simulink model "Control_Test"  (R2020a)
settings: Solver=ode1  StartTime=0.0  StopTime=inf  FixedStep=0.001  RelTol=1e-3
InitFcn:
  | COM_config;
  | IO_config;
values from neighbouring files (symbols this model uses):
  AirDensity_kgpm3 = 1.225    [vehicle_controller.mat]
  BatteryCapacity_Wh = 83    [vehicle_controller.mat]
  BatteryInitialEnergy = 58.1    [vehicle_controller.mat]
  BatteryMaxVoltage_V = 96    [vehicle_controller.mat]
  BatteryVoltageCoefficient_x = [0 0.1 0.2 0.3 0.4 0.5 0.6 0.7 0.8 0.9 1]    [vehicle_controller.mat]
  BatteryVoltageCoefficient_y = [0.833333333333 0.85 0.866666666667 0.883333333333 0.9 0.916666666667 0.933333333333 0.95 0.966666666667 0.983333333333 1]    [vehicle_controller.mat]
  BodyInitialSpeed_mps = 0    [vehicle_controller.mat]
  BodyMass_kg = 900    [vehicle_controller.mat]
  CombustionEngineMaxTorque_Nm = 100    [vehicle_controller.mat]
  DragArea_m2 = 4.5    [vehicle_controller.mat]
  DragCoeficient_1 = 0.4    [vehicle_controller.mat]
  FrictionCoefficient_Nsprad = 0.01    [vehicle_controller.mat]
  GearboxRatio_0_1 = 3    [vehicle_controller.mat]
  Ke = 0.1178    [vehicle_controller.mat]
  Kt = 0.668    [vehicle_controller.mat]
  L = looptransfer.Lo    [H_infinity_control_design.m]    (also in LoopShaping.m = G*K; Vehicle_Car_Controller.m = P * C)
  R = 0.141176    [vehicle_controller.mat]
  WheelDiameter_m = 0.5    [vehicle_controller.mat]
undefined symbols (not defined in the file or in its folder): AI_01_range, AI_02_range, AI_03_range, AI_04_range, AI_05_range, AI_06_range, AO_01_max, AO_02_max, AO_03_max, AO_04_max, AO_05_max, AO_06_max, Battery_Voltage_Req, DI_01_mode, DI_01_pullUpDown, DI_02_mode, DI_02_pullUpDown, DI_03_mode, DI_03_pullUpDown, DI_04_mode, DI_04_pullUpDown, DI_05_mode, DI_05_pullUpDown, DI_06_mode, DI_06_pullUpDown, DI_vref_threshold, DO_01_mode, DO_01_outStage, DO_02_mode, DO_02_outStage, DO_03_mode, DO_03_outStage, DO_04_mode, DO_04_outStage, DO_05_mode, DO_05_outStage, DO_06_mode, DO_06_outStage, DO_vref_high, package_period, Serial_Port, Standard_Devices
libraries: simulink x8, sldrtlib x2, simulink_extras x1
(part 1 of 2)
settings Model: SimulationMode=external  Creator=matti  LastModifiedBy=matti
settings SolverCC: DecoupledContinuousIntegration=on  MinimalZcImpactIntegration=on
settings DataIOCC: ReturnWorkspaceOutputs=off
settings DebuggingCC: ArithmeticOperatorsInVariantConditions=warning
settings SFSimCC: SimUseLocalCustomCode=off  CustomCodeUndefinedFunction=UseInterfaceOnly
settings RTWCC: Description=Simulink Desktop Real-Time  SystemTargetFile=sldrt.tlc  TemplateMakefile=sldrt.tmf  RTWUseLocalCustomCode=off  RTWCompilerOptimization=on
settings CodeAppCC: MaxIdLength=95
settings SimulinkDesktopRealTimeCC: TargetPreCompLibLocation=C:\Program Files\MATLAB\R2020a\toolbox\sldrt\lib\win64

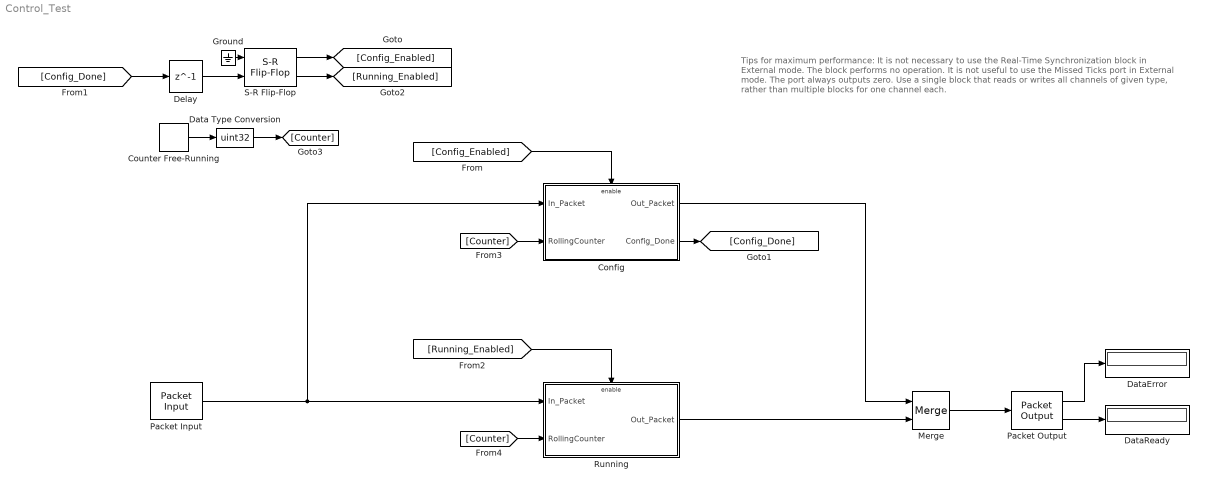
== system Control_Test ==
  note: Tips for maximum performance:
      |
      | It is not necessary to use the Real-Time Synchronization block in External mode. The block performs no operation.
      | It is not useful to use the Missed Ticks port in External mode. The port always outputs zero.
      | Use a single block that reads or writes all channels of given type, rather than multiple blocks for one channel each.
  Config : Subsystem
  Counter Free-Running : simulink/Sources/Counter Free-Running  NumBits=4  tsamp=package_period
  Data Type Conversion : DataTypeConversion  OutDataTypeStr=uint32
  DataError : Display
  DataReady : Display
  Delay : Delay  DelayLength=1  SampleTime=package_period
  Ground : Ground
  Merge : Merge  InitialOutput=uint32(zeros(1,64))
  Packet Input : sldrtlib/Packet Input  SampleTime=package_period  MaxMissedTicks=10  ShowMissedTicks=off  YieldWhenWaiting=off  DrvName=Standard_Devices/Serial_Port  DrvAddress=9  DrvOptions=[9600 8 0 0 0 0 0 0]  PacketSize=package_size  DataTypes=package_dataType  ShowReady=off  ShowError=off  PacketID=1  ByteOrder=1  ShowTimestamp=off
      settings: AttributesFormatString=Serial Port [9]
  Packet Output : sldrtlib/Packet Output  SampleTime=package_period  MaxMissedTicks=10  ShowMissedTicks=off  YieldWhenWaiting=off  DrvName=Standard_Devices/Serial_Port  DrvAddress=9  DrvOptions=[9600 8 0 0 0 0 0 0]  PacketSize=package_size  DataTypes=package_dataType  ShowReady=on  ShowError=on  PacketID=1  ByteOrder=1  InitialValue=[]  FinalValue=[]
      settings: AttributesFormatString=Serial Port [9]
  Running : Subsystem
  S-R Flip-Flop : simulink_extras/Flip Flops/S-R Flip-Flop  initial_condition=1
  wires:
  Packet Output/1 -> DataError/1
  Packet Output/2 -> DataReady/1
  Packet Input/1 -> Config/1(In_Packet), Running/1(In_Packet)
  Merge/1 -> Packet Output/1
  Running/1(Out_Packet) -> Merge/2
  [Config_Enabled] -> Config/Enable
  Config/2(Config_Done) -> [Config_Done]
  [Config_Done] -> Delay/1
  [Running_Enabled] -> Running/Enable
  S-R Flip-Flop/1 -> [Config_Enabled]
  S-R Flip-Flop/2 -> [Running_Enabled]
  Ground/1 -> S-R Flip-Flop/1
  Counter Free-Running/1 -> Data Type Conversion/1
  [Counter] -> Config/2(RollingCounter)
  [Counter] -> Running/2(RollingCounter)
  Data Type Conversion/1 -> [Counter]
  Delay/1 -> S-R Flip-Flop/2
  Config/1(Out_Packet) -> Merge/1

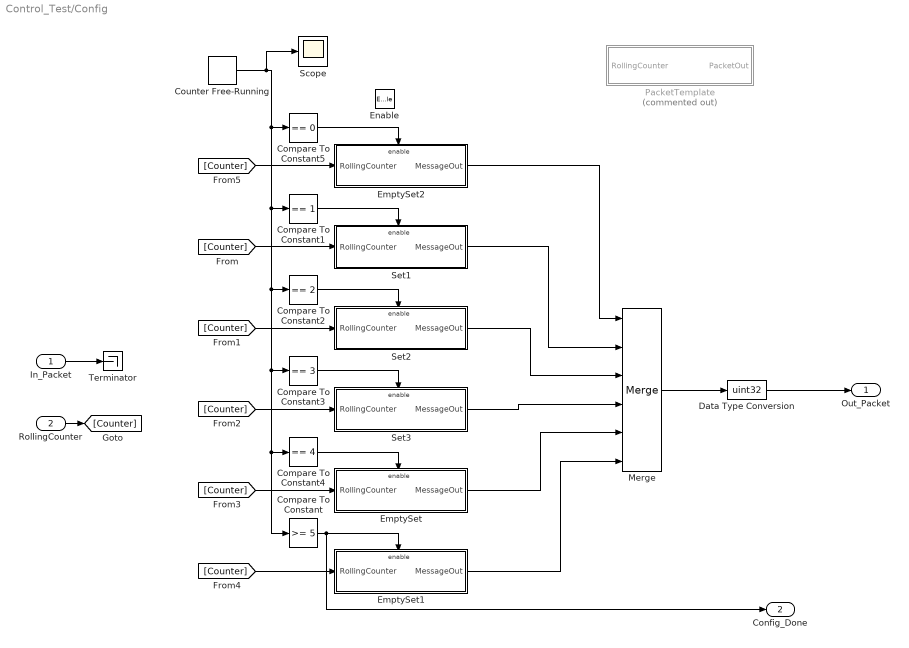
== system Control_Test/Config ==
  In_Packet : Inport
  RollingCounter : Inport  Port=2
  Enable : EnablePort
  Compare To Constant : simulink/Logic and Bit Operations/Compare To Constant  relop=>=  const=5  OutDataTypeStr=boolean
  Compare To Constant1 : simulink/Logic and Bit Operations/Compare To Constant  relop===  const=1  OutDataTypeStr=boolean
  Compare To Constant2 : simulink/Logic and Bit Operations/Compare To Constant  relop===  const=2  OutDataTypeStr=boolean
  Compare To Constant3 : simulink/Logic and Bit Operations/Compare To Constant  relop===  const=3  OutDataTypeStr=boolean
  Compare To Constant4 : simulink/Logic and Bit Operations/Compare To Constant  relop===  const=4  OutDataTypeStr=boolean
  Compare To Constant5 : simulink/Logic and Bit Operations/Compare To Constant  relop===  const=0  OutDataTypeStr=boolean
  Counter Free-Running : simulink/Sources/Counter Free-Running  NumBits=16  tsamp=package_period
  Data Type Conversion : DataTypeConversion  OutDataTypeStr=uint32
  EmptySet : Subsystem
  EmptySet1 : Subsystem
  EmptySet2 : Subsystem
  Merge : Merge  Inputs=6
  PacketTemplate : Subsystem  Commented=on
  Scope : Scope
  Set1 : Subsystem
  Set2 : Subsystem
  Set3 : Subsystem
  Terminator : Terminator
  Out_Packet : Outport
  Config_Done : Outport  Port=2
  wires:
  In_Packet/1 -> Terminator/1
  Compare To Constant/1 -> EmptySet1/Enable, Config_Done/1
  Counter Free-Running/1 -> Scope/1, Compare To Constant5/1, Compare To Constant/1, Compare To Constant4/1, Compare To Constant3/1, Compare To Constant2/1, Compare To Constant1/1
  Compare To Constant1/1 -> Set1/Enable
  Compare To Constant2/1 -> Set2/Enable
  Compare To Constant3/1 -> Set3/Enable
  Compare To Constant4/1 -> EmptySet/Enable
  Set1/1(MessageOut) -> Merge/2
  Set2/1(MessageOut) -> Merge/3
  Set3/1(MessageOut) -> Merge/4
  EmptySet/1(MessageOut) -> Merge/5
  EmptySet1/1(MessageOut) -> Merge/6
  RollingCounter/1 -> [Counter]
  [Counter] -> Set1/1(RollingCounter)
  [Counter] -> Set2/1(RollingCounter)
  [Counter] -> Set3/1(RollingCounter)
  [Counter] -> EmptySet/1(RollingCounter)
  [Counter] -> EmptySet1/1(RollingCounter)
  Merge/1 -> Data Type Conversion/1
  EmptySet2/1(MessageOut) -> Merge/1
  Compare To Constant5/1 -> EmptySet2/Enable
  [Counter] -> EmptySet2/1(RollingCounter)
  Data Type Conversion/1 -> Out_Packet/1

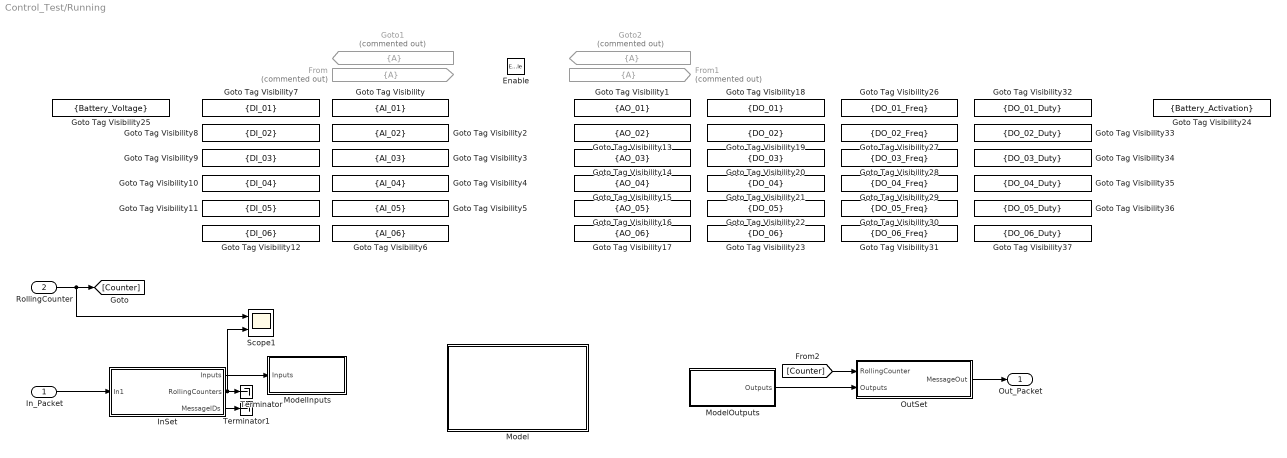
== system Control_Test/Running ==
  In_Packet : Inport
  RollingCounter : Inport  Port=2
  Enable : EnablePort
  From : From  Commented=on
  From1 : From  Commented=on
  Goto Tag Visibility : GotoTagVisibility  GotoTag=AI_01
  Goto Tag Visibility1 : GotoTagVisibility  GotoTag=AO_01
  Goto Tag Visibility10 : GotoTagVisibility  GotoTag=DI_04
  Goto Tag Visibility11 : GotoTagVisibility  GotoTag=DI_05
  Goto Tag Visibility12 : GotoTagVisibility  GotoTag=DI_06
  Goto Tag Visibility13 : GotoTagVisibility  GotoTag=AO_02
  Goto Tag Visibility14 : GotoTagVisibility  GotoTag=AO_03
  Goto Tag Visibility15 : GotoTagVisibility  GotoTag=AO_04
  Goto Tag Visibility16 : GotoTagVisibility  GotoTag=AO_05
  Goto Tag Visibility17 : GotoTagVisibility  GotoTag=AO_06
  Goto Tag Visibility18 : GotoTagVisibility  GotoTag=DO_01
  Goto Tag Visibility19 : GotoTagVisibility  GotoTag=DO_02
  Goto Tag Visibility2 : GotoTagVisibility  GotoTag=AI_02
  Goto Tag Visibility20 : GotoTagVisibility  GotoTag=DO_03
  Goto Tag Visibility21 : GotoTagVisibility  GotoTag=DO_04
  Goto Tag Visibility22 : GotoTagVisibility  GotoTag=DO_05
  Goto Tag Visibility23 : GotoTagVisibility  GotoTag=DO_06
  Goto Tag Visibility24 : GotoTagVisibility  GotoTag=Battery_Activation
  Goto Tag Visibility25 : GotoTagVisibility  GotoTag=Battery_Voltage
  Goto Tag Visibility26 : GotoTagVisibility  GotoTag=DO_01_Freq
  Goto Tag Visibility27 : GotoTagVisibility  GotoTag=DO_02_Freq
  Goto Tag Visibility28 : GotoTagVisibility  GotoTag=DO_03_Freq
  Goto Tag Visibility29 : GotoTagVisibility  GotoTag=DO_04_Freq
  Goto Tag Visibility3 : GotoTagVisibility  GotoTag=AI_03
  Goto Tag Visibility30 : GotoTagVisibility  GotoTag=DO_05_Freq
  Goto Tag Visibility31 : GotoTagVisibility  GotoTag=DO_06_Freq
  Goto Tag Visibility32 : GotoTagVisibility  GotoTag=DO_01_Duty
  Goto Tag Visibility33 : GotoTagVisibility  GotoTag=DO_02_Duty
  Goto Tag Visibility34 : GotoTagVisibility  GotoTag=DO_03_Duty
  Goto Tag Visibility35 : GotoTagVisibility  GotoTag=DO_04_Duty
  Goto Tag Visibility36 : GotoTagVisibility  GotoTag=DO_05_Duty
  Goto Tag Visibility37 : GotoTagVisibility  GotoTag=DO_06_Duty
  Goto Tag Visibility4 : GotoTagVisibility  GotoTag=AI_04
  Goto Tag Visibility5 : GotoTagVisibility  GotoTag=AI_05
  Goto Tag Visibility6 : GotoTagVisibility  GotoTag=AI_06
  Goto Tag Visibility7 : GotoTagVisibility  GotoTag=DI_01
  Goto Tag Visibility8 : GotoTagVisibility  GotoTag=DI_02
  Goto Tag Visibility9 : GotoTagVisibility  GotoTag=DI_03
  Goto1 : Goto  Commented=on  TagVisibility=scoped
  Goto2 : Goto  Commented=on  TagVisibility=scoped
  InSet : Subsystem
  Model : Subsystem
  ModelInputs : Subsystem
  ModelOutputs : Subsystem
  OutSet : Subsystem
  Scope1 : Scope  NumInputPorts=2
  Terminator : Terminator
  Terminator1 : Terminator
  Out_Packet : Outport
  wires:
  OutSet/1(MessageOut) -> Out_Packet/1
  ModelOutputs/1(Outputs) -> OutSet/2(Outputs)
  RollingCounter/1 -> Scope1/1, [Counter]
  [Counter] -> OutSet/1(RollingCounter)
  In_Packet/1 -> InSet/1(In1)
  InSet/1(Inputs) -> ModelInputs/1(Inputs)
  InSet/2(RollingCounters) -> Scope1/2, Terminator/1
  InSet/3(MessageIDs) -> Terminator1/1

== system Control_Test/Config/EmptySet ==
  RollingCounter : Inport
  Enable : EnablePort
  Empty1 : Subsystem
  Empty2 : Subsystem
  Empty3 : Subsystem
  Empty4 : Subsystem
  Empty5 : Subsystem
  Empty6 : Subsystem
  Empty7 : Subsystem
  Empty8 : Subsystem
  Mux : Mux  Inputs=8
  MessageOut : Outport
  wires:
  Mux/1 -> MessageOut/1
  Empty1/1(PacketOut) -> Mux/1
  Empty2/1(PacketOut) -> Mux/2
  Empty3/1(PacketOut) -> Mux/3
  Empty4/1(PacketOut) -> Mux/4
  Empty5/1(PacketOut) -> Mux/5
  Empty6/1(PacketOut) -> Mux/6
  Empty7/1(PacketOut) -> Mux/7
  Empty8/1(PacketOut) -> Mux/8
  RollingCounter/1 -> Empty1/1(RollingCounter), Empty2/1(RollingCounter), Empty3/1(RollingCounter), Empty4/1(RollingCounter), Empty5/1(RollingCounter), Empty6/1(RollingCounter), Empty8/1(RollingCounter), Empty7/1(RollingCounter)

== system Control_Test/Config/EmptySet1 ==
  RollingCounter : Inport
  Enable : EnablePort
  Empty1 : Subsystem
  Empty2 : Subsystem
  Empty3 : Subsystem
  Empty4 : Subsystem
  Empty5 : Subsystem
  Empty6 : Subsystem
  Empty7 : Subsystem
  Empty8 : Subsystem
  Mux : Mux  Inputs=8
  MessageOut : Outport
  wires:
  RollingCounter/1 -> Empty7/1(RollingCounter), Empty8/1(RollingCounter), Empty6/1(RollingCounter), Empty5/1(RollingCounter), Empty4/1(RollingCounter), Empty3/1(RollingCounter), Empty2/1(RollingCounter), Empty1/1(RollingCounter)
  Empty8/1(PacketOut) -> Mux/8
  Empty7/1(PacketOut) -> Mux/7
  Empty6/1(PacketOut) -> Mux/6
  Empty5/1(PacketOut) -> Mux/5
  Empty4/1(PacketOut) -> Mux/4
  Empty3/1(PacketOut) -> Mux/3
  Empty2/1(PacketOut) -> Mux/2
  Empty1/1(PacketOut) -> Mux/1
  Mux/1 -> MessageOut/1

== system Control_Test/Config/EmptySet2 ==
  RollingCounter : Inport
  Enable : EnablePort
  Empty1 : Subsystem
  Empty2 : Subsystem
  Empty3 : Subsystem
  Empty4 : Subsystem
  Empty5 : Subsystem
  Empty6 : Subsystem
  Empty7 : Subsystem
  Empty8 : Subsystem
  Mux : Mux  Inputs=8
  MessageOut : Outport
  wires:
  RollingCounter/1 -> Empty7/1(RollingCounter), Empty8/1(RollingCounter), Empty6/1(RollingCounter), Empty5/1(RollingCounter), Empty4/1(RollingCounter), Empty3/1(RollingCounter), Empty2/1(RollingCounter), Empty1/1(RollingCounter)
  Empty8/1(PacketOut) -> Mux/8
  Empty7/1(PacketOut) -> Mux/7
  Empty6/1(PacketOut) -> Mux/6
  Empty5/1(PacketOut) -> Mux/5
  Empty4/1(PacketOut) -> Mux/4
  Empty3/1(PacketOut) -> Mux/3
  Empty2/1(PacketOut) -> Mux/2
  Empty1/1(PacketOut) -> Mux/1
  Mux/1 -> MessageOut/1

== system Control_Test/Config/PacketTemplate ==
  RollingCounter : Inport
  Data{1..6} (6 alike) : Constant  Value=0
  ID : Constant  Value=0
  Mux : Mux  Inputs=8
  PacketOut : Outport
  wires:
  Mux/1 -> PacketOut/1
  ID/1 -> Mux/1
  Data1/1 -> Mux/2
  Data2/1 -> Mux/3
  Data3/1 -> Mux/4
  Data4/1 -> Mux/5
  Data5/1 -> Mux/6
  Data6/1 -> Mux/7
  RollingCounter/1 -> Mux/8

== system Control_Test/Config/Set1 ==
  RollingCounter : Inport
  Enable : EnablePort
  0x1011 : Subsystem
  Empty1 : Subsystem
  Empty2 : Subsystem
  Empty3 : Subsystem
  Empty4 : Subsystem
  Empty5 : Subsystem
  Empty6 : Subsystem
  Empty7 : Subsystem
  Mux : Mux  Inputs=8
  MessageOut : Outport
  wires:
  Mux/1 -> MessageOut/1
  0x1011/1(PacketOut) -> Mux/1
  Empty1/1(PacketOut) -> Mux/2
  Empty2/1(PacketOut) -> Mux/3
  Empty3/1(PacketOut) -> Mux/4
  Empty4/1(PacketOut) -> Mux/5
  Empty5/1(PacketOut) -> Mux/6
  Empty6/1(PacketOut) -> Mux/7
  Empty7/1(PacketOut) -> Mux/8
  RollingCounter/1 -> Empty1/1(RollingCounter), Empty2/1(RollingCounter), Empty3/1(RollingCounter), Empty4/1(RollingCounter), Empty5/1(RollingCounter), Empty7/1(RollingCounter), Empty6/1(RollingCounter), 0x1011/1(RollingCounter)

== system Control_Test/Config/Set2 ==
  RollingCounter : Inport
  Enable : EnablePort
  0x1012 : Subsystem
  0x1013 : Subsystem
  0x1029 : Subsystem
  0x1039 : Subsystem
  0x1047 : Subsystem
  0x1048 : Subsystem
  0x1049 : Subsystem
  0x1058 : Subsystem
  Mux : Mux  Inputs=8
  MessageOut : Outport
  wires:
  0x1058/1(PacketOut) -> Mux/8
  0x1047/1(PacketOut) -> Mux/5
  0x1049/1(PacketOut) -> Mux/7
  0x1039/1(PacketOut) -> Mux/4
  0x1013/1(PacketOut) -> Mux/2
  RollingCounter/1 -> 0x1013/1(RollingCounter), 0x1029/1(RollingCounter), 0x1039/1(RollingCounter), 0x1047/1(RollingCounter), 0x1048/1(RollingCounter), 0x1049/1(RollingCounter), 0x1058/1(RollingCounter), 0x1012/1(RollingCounter)
  0x1012/1(PacketOut) -> Mux/1
  Mux/1 -> MessageOut/1
  0x1029/1(PacketOut) -> Mux/3
  0x1048/1(PacketOut) -> Mux/6

== system Control_Test/Config/Set3 ==
  RollingCounter : Inport
  Enable : EnablePort
  0x1057 : Subsystem
  0x1059 : Subsystem
  Empty2 : Subsystem
  Empty3 : Subsystem
  Empty4 : Subsystem
  Empty5 : Subsystem
  Empty6 : Subsystem
  Empty7 : Subsystem
  Mux : Mux  Inputs=8
  MessageOut : Outport
  wires:
  RollingCounter/1 -> 0x1059/1(RollingCounter), 0x1057/1(RollingCounter), Empty2/1(RollingCounter), Empty3/1(RollingCounter), Empty4/1(RollingCounter), Empty5/1(RollingCounter), Empty7/1(RollingCounter), Empty6/1(RollingCounter)
  Empty7/1(PacketOut) -> Mux/8
  Empty6/1(PacketOut) -> Mux/7
  Empty5/1(PacketOut) -> Mux/6
  Empty4/1(PacketOut) -> Mux/5
  Empty3/1(PacketOut) -> Mux/4
  Empty2/1(PacketOut) -> Mux/3
  0x1057/1(PacketOut) -> Mux/2
  0x1059/1(PacketOut) -> Mux/1
  Mux/1 -> MessageOut/1

== system Control_Test/Running/InSet ==
  In1 : Inport
  AI : Subsystem
  BatteryVoltage : Subsystem
  Bus Creator : BusCreator  Inputs=3
  DI : Subsystem
  Demux1 : Demux  Outputs=8
  Empty2 : Subsystem
  Empty3 : Subsystem
  Empty4 : Subsystem
  Empty5 : Subsystem
  Empty6 : Subsystem
  Mux : Mux  Inputs=8.
  Mux1 : Mux  Inputs=8.
  Inputs : Outport
  RollingCounters : Outport  Port=2
  MessageIDs : Outport  Port=3
  wires:
  Demux1/6 -> Empty3/1(PacketIn)
  Demux1/4 -> BatteryVoltage/1(PacketIn)
  AI/3(AI) -> Bus Creator/1  "AI"
  Demux1/2 -> AI/1(PacketIn)
  Empty4/2(ID) -> Mux/7
  Demux1/3 -> DI/1(PacketIn)
  BatteryVoltage/1(RollingCounter) -> Mux1/4
  Demux1/8 -> Empty5/1(PacketIn)
  Empty2/1(RollingCounter) -> Mux1/5
  Empty5/1(RollingCounter) -> Mux1/8
  Empty4/1(RollingCounter) -> Mux1/7
  Empty3/1(RollingCounter) -> Mux1/6
  Empty2/2(ID) -> Mux/5
  Demux1/5 -> Empty2/1(PacketIn)
  Empty3/2(ID) -> Mux/6
  DI/3(DI) -> Bus Creator/2  "DI"
  Demux1/7 -> Empty4/1(PacketIn)
  BatteryVoltage/2(ID) -> Mux/4
  In1/1 -> Demux1/1
  Empty5/2(ID) -> Mux/8
  Demux1/1 -> Empty6/1(PacketIn)
  Mux1/1 -> RollingCounters/1
  Mux/1 -> MessageIDs/1
  Bus Creator/1 -> Inputs/1
  DI/1(RollingCounter) -> Mux1/3
  DI/2(ID) -> Mux/3
  AI/2(ID) -> Mux/2
  AI/1(RollingCounter) -> Mux1/2
  Empty6/1(RollingCounter) -> Mux1/1
  Empty6/2(ID) -> Mux/1
  BatteryVoltage/3(Battery_Voltage) -> Bus Creator/3  "Battery_Voltage"

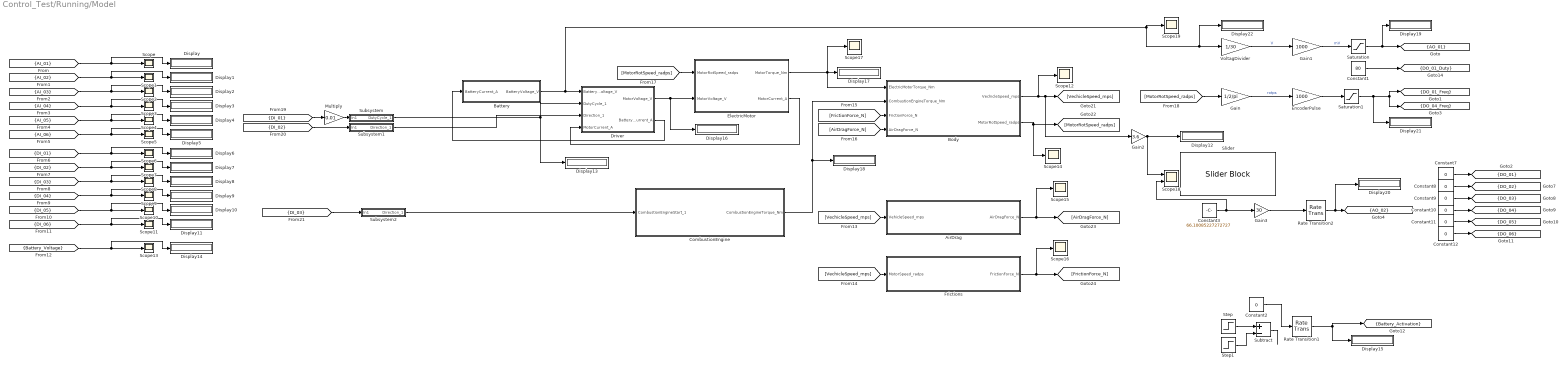
== system Control_Test/Running/Model ==
  AirDrag : Subsystem
  Battery : Subsystem
  Body : Subsystem
  CombustionEngine : Subsystem
  Constant1 : Constant  Value=80
  Constant{2,7..12} (7 alike) : Constant  Value=0
  Constant3 : Constant  Value=66.10085227272727  OutDataTypeStr=Inherit: Inherit via back propagation
  Display{,1..22} (23 alike) : Display
  Driver : Subsystem
  ElectricMotor : Subsystem
  EncoderPulse : Gain  Gain=1000
  Frictions : Subsystem
  Gain : Gain  Gain=1/2/pi
  Gain1 : Gain  Gain=1000
  Gain2 : Gain  Gain=3.6
  Gain3 : Gain  Gain=30
  Multiply : Gain  Gain=0.01
  Rate Transition1 : RateTransition
  Rate Transition2 : RateTransition
  Saturation : Saturate  UpperLimit=3300  LowerLimit=1
  Saturation1 : Saturate  UpperLimit=100000  LowerLimit=1
  Scope{,1..17,19} (19 alike) : Scope
  Scope18 : Scope  NumInputPorts=2
  Slider : SliderBlock
  Step : Step  Time=10  SampleTime=0
  Step1 : Step  Time=59.9  SampleTime=0
  Subsystem : Subsystem
  Subsystem1 : Subsystem
  Subsystem2 : Subsystem
  Subtract : Sum  Inputs=+-
  VoltagDivider : Gain  Gain=1/30
  tag scope: AO_01=scoped, AO_02=scoped, Battery_Activation=scoped, DO_01=scoped, DO_01_Duty=scoped, DO_01_Freq=scoped, DO_02=scoped, DO_03=scoped, DO_04=scoped, DO_04_Freq=scoped, DO_05=scoped, DO_06=scoped
  wires:
  [AI_01] -> Display/1, Scope/1
  [AI_02] -> Display1/1, Scope1/1
  [AI_03] -> Display2/1, Scope2/1
  [AI_04] -> Display3/1, Scope3/1
  [AI_05] -> Display4/1, Scope4/1
  [AI_06] -> Display5/1, Scope5/1
  [DI_01] -> Display6/1, Scope6/1
  [DI_02] -> Display7/1, Scope7/1
  [DI_03] -> Display8/1, Scope8/1
  [DI_04] -> Display9/1, Scope9/1
  [DI_05] -> Display10/1, Scope10/1
  [DI_06] -> Display11/1, Scope11/1
  Constant7/1 -> [DO_01]
  Constant8/1 -> [DO_02]
  Constant9/1 -> [DO_03]
  Constant10/1 -> [DO_04]
  Constant11/1 -> [DO_05]
  Constant12/1 -> [DO_06]
  [Battery_Voltage] -> Scope13/1, Display14/1
  Subtract/1 -> ?
  Rate Transition1/1 -> [Battery_Activation], Display15/1
  Step/1 -> Subtract/1
  Step1/1 -> Subtract/2
  Constant2/1 -> Rate Transition1/1
  Gain1/1 -> Saturation/1  "mV"
  Constant1/1 -> [DO_01_Duty]
  Driver/1(MotorVoltage_V) -> Display16/1, ElectricMotor/2(MotorVoltage_V)
  Body/1(VechicleSpeed_mps) -> Gain2/1, [VechicleSpeed_mps], Scope12/1
  ElectricMotor/1(MotorTorque_Nm) -> Scope17/1, Display17/1, Body/1(ElectricMotorTorque_Nm)
  Body/2(MotorRotSpeed_radps) -> Scope14/1, [MotorRotSpeed_radps]
  Frictions/1(FrictionForce_N) -> Scope16/1, [FrictionForce_N]
  AirDrag/1(AirDragForce_N) -> [AirDragForce_N], Scope15/1
  CombustionEngine/1(CombustionEngineTorque_Nm) -> Display18/1, Body/2(CombustionEngineTorque_Nm)
  [VechicleSpeed_mps] -> AirDrag/1(VehicleSpeed_mps)
  [VechicleSpeed_mps] -> Frictions/1(MotorSpeed_radps)
  [FrictionForce_N] -> Body/3(FrictionForce_N)
  [AirDragForce_N] -> Body/4(AirDragForce_N)
  [MotorRotSpeed_radps] -> ElectricMotor/1(MotorRotSpeed_radps)
  Battery/1(BatteryVoltage_V) -> Display22/1, VoltagDivider/1, Scope19/1, Driver/1(BatteryVoltage_V)
  Driver/2(BatteryCurrent_A) -> Battery/1(BatteryCurrent_A)
  ElectricMotor/2(MotorCurrent_A) -> Driver/4(MotorCurrent_A)
  EncoderPulse/1 -> Saturation1/1
  [MotorRotSpeed_radps] -> Gain/1
  Gain/1 -> EncoderPulse/1  "rotps"
  VoltagDivider/1 -> Gain1/1  "V"
  Saturation/1 -> Display19/1, [AO_01]
  Subsystem1/1(Direction_1) -> Driver/3(Direction_1)
  [DI_03] -> Subsystem2/1(In1)
  Saturation1/1 -> Display21/1, [DO_01_Freq], [DO_04_Freq]
  Gain2/1 -> Scope18/1, Display12/1
  Constant3/1 -> Scope18/2, Gain3/1
  Rate Transition2/1 -> Display20/1, [AO_02]
  Gain3/1 -> Rate Transition2/1
  Subsystem/1(DutyCycle_1) -> Driver/2(DutyCycle_1), Display13/1
  [DI_01] -> Multiply/1
  [DI_02] -> Subsystem1/1(In1)
  Subsystem2/1(Direction_1) -> CombustionEngine/1(CombustionEngineStart_1)
  Multiply/1 -> Subsystem/1(In1)

== system Control_Test/Running/ModelInputs ==
  Inputs : Inport
  Bus Selector : BusSelector  OutputSignals=AI,DI,Battery_Voltage
  Data Type Conversion : DataTypeConversion
  Subsystem2 : Subsystem
  Subsystem3 : Subsystem
  tag scope: Battery_Voltage=scoped
  wires:
  Bus Selector/1 -> Subsystem2/1(<AI>)  "<AI>"
  Bus Selector/2 -> Subsystem3/1(<DI>)  "<DI>"
  Inputs/1 -> Bus Selector/1
  Data Type Conversion/1 -> [Battery_Voltage]
  Bus Selector/3 -> Data Type Conversion/1  "<Battery_Voltage>"

== system Control_Test/Running/ModelOutputs ==
  AO : Subsystem
  Bus Creator4 : BusCreator  Inputs=5
  DO_Duty : Subsystem
  DO_Freq : Subsystem
  DO_Level : Subsystem
  Data Type Conversion : DataTypeConversion  OutDataTypeStr=uint32
  Rate Transition1 : RateTransition
  Outputs : Outport
  wires:
  AO/1(AO) -> Bus Creator4/1  "AO"
  DO_Level/1(DO_Level) -> Bus Creator4/2  "DO_Level"
  DO_Freq/1(DO_Freq) -> Bus Creator4/3  "DO_Freq"
  DO_Duty/1(DO_Duty) -> Bus Creator4/4  "DO_Duty"
  Bus Creator4/1 -> Rate Transition1/1
  Data Type Conversion/1 -> Bus Creator4/5  "Battery_Activation"
  [Battery_Activation] -> Data Type Conversion/1  "Battery_Activation"
  Rate Transition1/1 -> Outputs/1

== system Control_Test/Running/OutSet ==
  RollingCounter : Inport
  Outputs : Inport  Port=2
  0x1019 : Subsystem
  0x1031 : Subsystem
  0x1051 : Subsystem
  0x1052 : Subsystem
  0x1053 : Subsystem
  Bus Selector : BusSelector  OutputSignals=AO,DO_Level,DO_Freq,DO_Duty,Battery_Activation
  Empty2 : Subsystem
  Empty3 : Subsystem
  Empty4 : Subsystem
  Mux : Mux  Inputs=8
  MessageOut : Outport
  wires:
  0x1031/1(PacketOut) -> Mux/1
  0x1051/1(PacketOut) -> Mux/2
  0x1052/1(PacketOut) -> Mux/3
  0x1053/1(PacketOut) -> Mux/4
  0x1019/1(PacketOut) -> Mux/5
  Empty2/1(PacketOut) -> Mux/6
  Empty3/1(PacketOut) -> Mux/7
  Empty4/1(PacketOut) -> Mux/8
  RollingCounter/1 -> Empty2/1(RollingCounter), Empty4/1(RollingCounter), Empty3/1(RollingCounter), 0x1019/1(RollingCounter), 0x1053/1(RollingCounter), 0x1052/1(RollingCounter), 0x1051/1(RollingCounter), 0x1031/1(RollingCounter)
  Bus Selector/1 -> 0x1031/2(DAC)  "<AO>"
  Bus Selector/2 -> 0x1051/2(DO_Level)  "<DO_Level>"
  Bus Selector/3 -> 0x1052/2(DO_Freq)  "<DO_Freq>"
  Bus Selector/4 -> 0x1053/2(DO_Duty)  "<DO_Duty>"
  Outputs/1 -> Bus Selector/1
  Mux/1 -> MessageOut/1
  Bus Selector/5 -> 0x1019/2(Battery_Active)  "<Battery_Activation>"

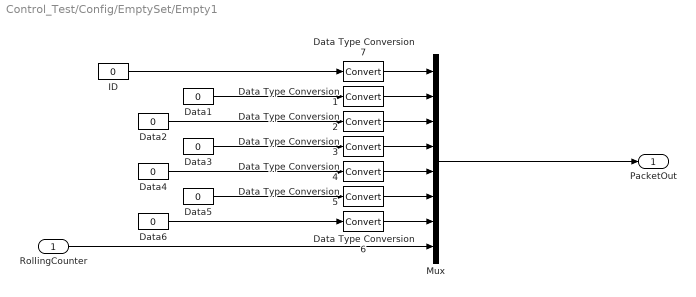
== system Control_Test/Config/EmptySet/Empty1 ==
  RollingCounter : Inport
  Data Type Conversion{1..7} (7 alike) : DataTypeConversion
  Data{1..6} (6 alike) : Constant  Value=0
  ID : Constant  Value=0
  Mux : Mux  Inputs=8
  PacketOut : Outport
  wires:
  RollingCounter/1 -> Mux/8
  Data6/1 -> Data Type Conversion6/1
  Data5/1 -> Data Type Conversion5/1
  Data4/1 -> Data Type Conversion4/1
  Data3/1 -> Data Type Conversion3/1
  Data2/1 -> Data Type Conversion2/1
  Data1/1 -> Data Type Conversion1/1
  ID/1 -> Data Type Conversion7/1
  Mux/1 -> PacketOut/1
  Data Type Conversion4/1 -> Mux/5
  Data Type Conversion6/1 -> Mux/7
  Data Type Conversion2/1 -> Mux/3
  Data Type Conversion1/1 -> Mux/2
  Data Type Conversion3/1 -> Mux/4
  Data Type Conversion5/1 -> Mux/6
  Data Type Conversion7/1 -> Mux/1

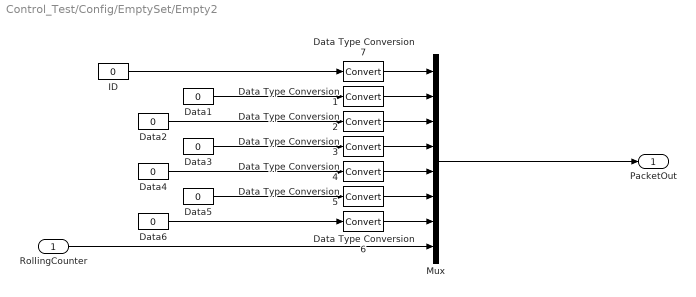
== system Control_Test/Config/EmptySet/Empty2 ==
  RollingCounter : Inport
  Data Type Conversion{1..7} (7 alike) : DataTypeConversion
  Data{1..6} (6 alike) : Constant  Value=0
  ID : Constant  Value=0
  Mux : Mux  Inputs=8
  PacketOut : Outport
  wires:
  Data Type Conversion7/1 -> Mux/1
  Data Type Conversion5/1 -> Mux/6
  Data Type Conversion3/1 -> Mux/4
  Data Type Conversion1/1 -> Mux/2
  Data Type Conversion2/1 -> Mux/3
  Data Type Conversion6/1 -> Mux/7
  Data Type Conversion4/1 -> Mux/5
  Mux/1 -> PacketOut/1
  ID/1 -> Data Type Conversion7/1
  Data1/1 -> Data Type Conversion1/1
  Data2/1 -> Data Type Conversion2/1
  Data3/1 -> Data Type Conversion3/1
  Data4/1 -> Data Type Conversion4/1
  Data5/1 -> Data Type Conversion5/1
  Data6/1 -> Data Type Conversion6/1
  RollingCounter/1 -> Mux/8

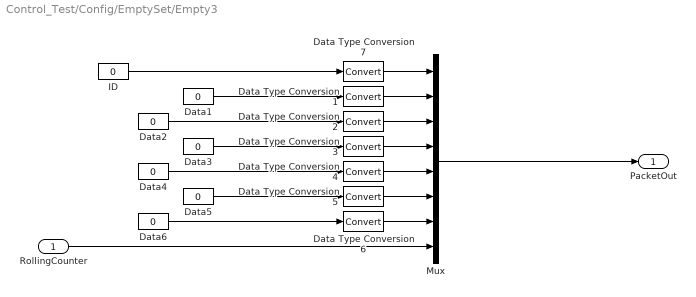
== system Control_Test/Config/EmptySet/Empty3 ==
  RollingCounter : Inport
  Data Type Conversion{1..7} (7 alike) : DataTypeConversion
  Data{1..6} (6 alike) : Constant  Value=0
  ID : Constant  Value=0
  Mux : Mux  Inputs=8
  PacketOut : Outport
  wires:
  Data Type Conversion7/1 -> Mux/1
  Data Type Conversion5/1 -> Mux/6
  Data Type Conversion3/1 -> Mux/4
  Data Type Conversion1/1 -> Mux/2
  Data Type Conversion2/1 -> Mux/3
  Data Type Conversion6/1 -> Mux/7
  Data Type Conversion4/1 -> Mux/5
  Mux/1 -> PacketOut/1
  ID/1 -> Data Type Conversion7/1
  Data1/1 -> Data Type Conversion1/1
  Data2/1 -> Data Type Conversion2/1
  Data3/1 -> Data Type Conversion3/1
  Data4/1 -> Data Type Conversion4/1
  Data5/1 -> Data Type Conversion5/1
  Data6/1 -> Data Type Conversion6/1
  RollingCounter/1 -> Mux/8

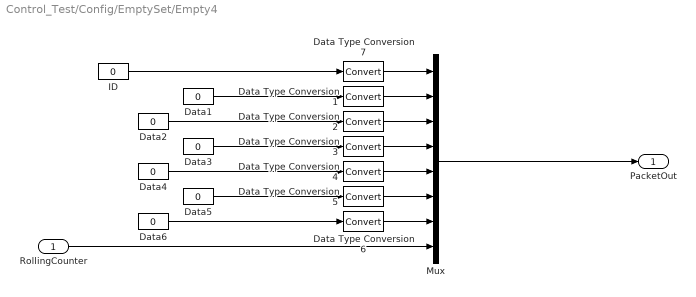
== system Control_Test/Config/EmptySet/Empty4 ==
  RollingCounter : Inport
  Data Type Conversion{1..7} (7 alike) : DataTypeConversion
  Data{1..6} (6 alike) : Constant  Value=0
  ID : Constant  Value=0
  Mux : Mux  Inputs=8
  PacketOut : Outport
  wires:
  RollingCounter/1 -> Mux/8
  Data6/1 -> Data Type Conversion6/1
  Data5/1 -> Data Type Conversion5/1
  Data4/1 -> Data Type Conversion4/1
  Data3/1 -> Data Type Conversion3/1
  Data2/1 -> Data Type Conversion2/1
  Data1/1 -> Data Type Conversion1/1
  ID/1 -> Data Type Conversion7/1
  Mux/1 -> PacketOut/1
  Data Type Conversion4/1 -> Mux/5
  Data Type Conversion6/1 -> Mux/7
  Data Type Conversion2/1 -> Mux/3
  Data Type Conversion1/1 -> Mux/2
  Data Type Conversion3/1 -> Mux/4
  Data Type Conversion5/1 -> Mux/6
  Data Type Conversion7/1 -> Mux/1

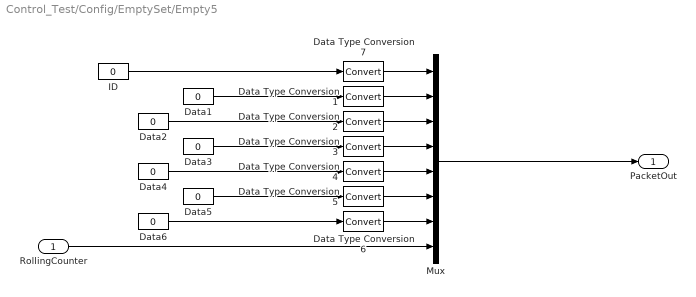
== system Control_Test/Config/EmptySet/Empty5 ==
  RollingCounter : Inport
  Data Type Conversion{1..7} (7 alike) : DataTypeConversion
  Data{1..6} (6 alike) : Constant  Value=0
  ID : Constant  Value=0
  Mux : Mux  Inputs=8
  PacketOut : Outport
  wires:
  Data Type Conversion7/1 -> Mux/1
  Data Type Conversion5/1 -> Mux/6
  Data Type Conversion3/1 -> Mux/4
  Data Type Conversion1/1 -> Mux/2
  Data Type Conversion2/1 -> Mux/3
  Data Type Conversion6/1 -> Mux/7
  Data Type Conversion4/1 -> Mux/5
  Mux/1 -> PacketOut/1
  ID/1 -> Data Type Conversion7/1
  Data1/1 -> Data Type Conversion1/1
  Data2/1 -> Data Type Conversion2/1
  Data3/1 -> Data Type Conversion3/1
  Data4/1 -> Data Type Conversion4/1
  Data5/1 -> Data Type Conversion5/1
  Data6/1 -> Data Type Conversion6/1
  RollingCounter/1 -> Mux/8

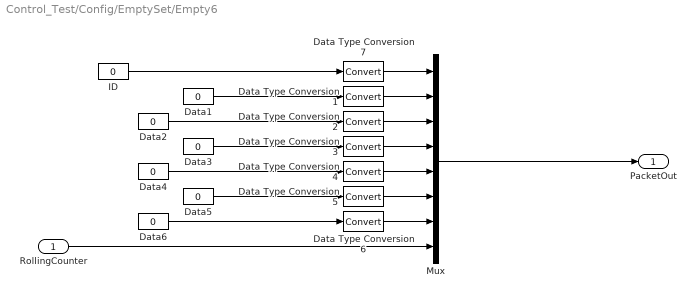
== system Control_Test/Config/EmptySet/Empty6 ==
  RollingCounter : Inport
  Data Type Conversion{1..7} (7 alike) : DataTypeConversion
  Data{1..6} (6 alike) : Constant  Value=0
  ID : Constant  Value=0
  Mux : Mux  Inputs=8
  PacketOut : Outport
  wires:
  RollingCounter/1 -> Mux/8
  Data6/1 -> Data Type Conversion6/1
  Data5/1 -> Data Type Conversion5/1
  Data4/1 -> Data Type Conversion4/1
  Data3/1 -> Data Type Conversion3/1
  Data2/1 -> Data Type Conversion2/1
  Data1/1 -> Data Type Conversion1/1
  ID/1 -> Data Type Conversion7/1
  Mux/1 -> PacketOut/1
  Data Type Conversion4/1 -> Mux/5
  Data Type Conversion6/1 -> Mux/7
  Data Type Conversion2/1 -> Mux/3
  Data Type Conversion1/1 -> Mux/2
  Data Type Conversion3/1 -> Mux/4
  Data Type Conversion5/1 -> Mux/6
  Data Type Conversion7/1 -> Mux/1

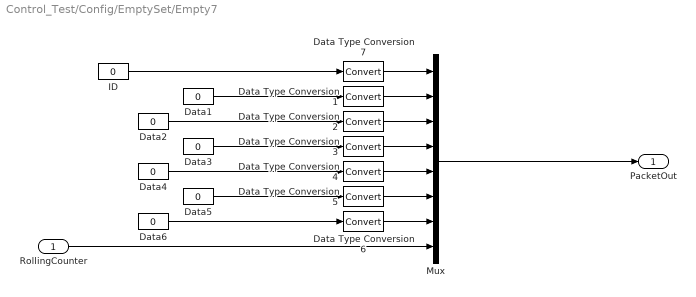
== system Control_Test/Config/EmptySet/Empty7 ==
  RollingCounter : Inport
  Data Type Conversion{1..7} (7 alike) : DataTypeConversion
  Data{1..6} (6 alike) : Constant  Value=0
  ID : Constant  Value=0
  Mux : Mux  Inputs=8
  PacketOut : Outport
  wires:
  RollingCounter/1 -> Mux/8
  Data6/1 -> Data Type Conversion6/1
  Data5/1 -> Data Type Conversion5/1
  Data4/1 -> Data Type Conversion4/1
  Data3/1 -> Data Type Conversion3/1
  Data2/1 -> Data Type Conversion2/1
  Data1/1 -> Data Type Conversion1/1
  ID/1 -> Data Type Conversion7/1
  Mux/1 -> PacketOut/1
  Data Type Conversion4/1 -> Mux/5
  Data Type Conversion6/1 -> Mux/7
  Data Type Conversion2/1 -> Mux/3
  Data Type Conversion1/1 -> Mux/2
  Data Type Conversion3/1 -> Mux/4
  Data Type Conversion5/1 -> Mux/6
  Data Type Conversion7/1 -> Mux/1

== system Control_Test/Config/EmptySet/Empty8 ==
  RollingCounter : Inport
  Data Type Conversion{1..7} (7 alike) : DataTypeConversion
  Data{1..6} (6 alike) : Constant  Value=0
  ID : Constant  Value=0
  Mux : Mux  Inputs=8
  PacketOut : Outport
  wires:
  Data Type Conversion7/1 -> Mux/1
  Data Type Conversion5/1 -> Mux/6
  Data Type Conversion3/1 -> Mux/4
  Data Type Conversion1/1 -> Mux/2
  Data Type Conversion2/1 -> Mux/3
  Data Type Conversion6/1 -> Mux/7
  Data Type Conversion4/1 -> Mux/5
  Mux/1 -> PacketOut/1
  ID/1 -> Data Type Conversion7/1
  Data1/1 -> Data Type Conversion1/1
  Data2/1 -> Data Type Conversion2/1
  Data3/1 -> Data Type Conversion3/1
  Data4/1 -> Data Type Conversion4/1
  Data5/1 -> Data Type Conversion5/1
  Data6/1 -> Data Type Conversion6/1
  RollingCounter/1 -> Mux/8

== system Control_Test/Config/EmptySet1/Empty1 ==
  RollingCounter : Inport
  Data Type Conversion{1..7} (7 alike) : DataTypeConversion
  Data{1..6} (6 alike) : Constant  Value=0
  ID : Constant  Value=0
  Mux : Mux  Inputs=8
  PacketOut : Outport
  wires:
  Data Type Conversion7/1 -> Mux/1
  Data Type Conversion5/1 -> Mux/6
  Data Type Conversion3/1 -> Mux/4
  Data Type Conversion1/1 -> Mux/2
  Data Type Conversion2/1 -> Mux/3
  Data Type Conversion6/1 -> Mux/7
  Data Type Conversion4/1 -> Mux/5
  Mux/1 -> PacketOut/1
  ID/1 -> Data Type Conversion7/1
  Data1/1 -> Data Type Conversion1/1
  Data2/1 -> Data Type Conversion2/1
  Data3/1 -> Data Type Conversion3/1
  Data4/1 -> Data Type Conversion4/1
  Data5/1 -> Data Type Conversion5/1
  Data6/1 -> Data Type Conversion6/1
  RollingCounter/1 -> Mux/8

== system Control_Test/Config/EmptySet1/Empty2 ==
  RollingCounter : Inport
  Data Type Conversion{1..7} (7 alike) : DataTypeConversion
  Data{1..6} (6 alike) : Constant  Value=0
  ID : Constant  Value=0
  Mux : Mux  Inputs=8
  PacketOut : Outport
  wires:
  RollingCounter/1 -> Mux/8
  Data6/1 -> Data Type Conversion6/1
  Data5/1 -> Data Type Conversion5/1
  Data4/1 -> Data Type Conversion4/1
  Data3/1 -> Data Type Conversion3/1
  Data2/1 -> Data Type Conversion2/1
  Data1/1 -> Data Type Conversion1/1
  ID/1 -> Data Type Conversion7/1
  Mux/1 -> PacketOut/1
  Data Type Conversion4/1 -> Mux/5
  Data Type Conversion6/1 -> Mux/7
  Data Type Conversion2/1 -> Mux/3
  Data Type Conversion1/1 -> Mux/2
  Data Type Conversion3/1 -> Mux/4
  Data Type Conversion5/1 -> Mux/6
  Data Type Conversion7/1 -> Mux/1

== system Control_Test/Config/EmptySet1/Empty3 ==
  RollingCounter : Inport
  Data Type Conversion{1..7} (7 alike) : DataTypeConversion
  Data{1..6} (6 alike) : Constant  Value=0
  ID : Constant  Value=0
  Mux : Mux  Inputs=8
  PacketOut : Outport
  wires:
  RollingCounter/1 -> Mux/8
  Data6/1 -> Data Type Conversion6/1
  Data5/1 -> Data Type Conversion5/1
  Data4/1 -> Data Type Conversion4/1
  Data3/1 -> Data Type Conversion3/1
  Data2/1 -> Data Type Conversion2/1
  Data1/1 -> Data Type Conversion1/1
  ID/1 -> Data Type Conversion7/1
  Mux/1 -> PacketOut/1
  Data Type Conversion4/1 -> Mux/5
  Data Type Conversion6/1 -> Mux/7
  Data Type Conversion2/1 -> Mux/3
  Data Type Conversion1/1 -> Mux/2
  Data Type Conversion3/1 -> Mux/4
  Data Type Conversion5/1 -> Mux/6
  Data Type Conversion7/1 -> Mux/1

== system Control_Test/Config/EmptySet1/Empty4 ==
  RollingCounter : Inport
  Data Type Conversion{1..7} (7 alike) : DataTypeConversion
  Data{1..6} (6 alike) : Constant  Value=0
  ID : Constant  Value=0
  Mux : Mux  Inputs=8
  PacketOut : Outport
  wires:
  Data Type Conversion7/1 -> Mux/1
  Data Type Conversion5/1 -> Mux/6
  Data Type Conversion3/1 -> Mux/4
  Data Type Conversion1/1 -> Mux/2
  Data Type Conversion2/1 -> Mux/3
  Data Type Conversion6/1 -> Mux/7
  Data Type Conversion4/1 -> Mux/5
  Mux/1 -> PacketOut/1
  ID/1 -> Data Type Conversion7/1
  Data1/1 -> Data Type Conversion1/1
  Data2/1 -> Data Type Conversion2/1
  Data3/1 -> Data Type Conversion3/1
  Data4/1 -> Data Type Conversion4/1
  Data5/1 -> Data Type Conversion5/1
  Data6/1 -> Data Type Conversion6/1
  RollingCounter/1 -> Mux/8

== system Control_Test/Config/EmptySet1/Empty5 ==
  RollingCounter : Inport
  Data Type Conversion{1..7} (7 alike) : DataTypeConversion
  Data{1..6} (6 alike) : Constant  Value=0
  ID : Constant  Value=0
  Mux : Mux  Inputs=8
  PacketOut : Outport
  wires:
  RollingCounter/1 -> Mux/8
  Data6/1 -> Data Type Conversion6/1
  Data5/1 -> Data Type Conversion5/1
  Data4/1 -> Data Type Conversion4/1
  Data3/1 -> Data Type Conversion3/1
  Data2/1 -> Data Type Conversion2/1
  Data1/1 -> Data Type Conversion1/1
  ID/1 -> Data Type Conversion7/1
  Mux/1 -> PacketOut/1
  Data Type Conversion4/1 -> Mux/5
  Data Type Conversion6/1 -> Mux/7
  Data Type Conversion2/1 -> Mux/3
  Data Type Conversion1/1 -> Mux/2
  Data Type Conversion3/1 -> Mux/4
  Data Type Conversion5/1 -> Mux/6
  Data Type Conversion7/1 -> Mux/1

== system Control_Test/Config/EmptySet1/Empty6 ==
  RollingCounter : Inport
  Data Type Conversion{1..7} (7 alike) : DataTypeConversion
  Data{1..6} (6 alike) : Constant  Value=0
  ID : Constant  Value=0
  Mux : Mux  Inputs=8
  PacketOut : Outport
  wires:
  Data Type Conversion7/1 -> Mux/1
  Data Type Conversion5/1 -> Mux/6
  Data Type Conversion3/1 -> Mux/4
  Data Type Conversion1/1 -> Mux/2
  Data Type Conversion2/1 -> Mux/3
  Data Type Conversion6/1 -> Mux/7
  Data Type Conversion4/1 -> Mux/5
  Mux/1 -> PacketOut/1
  ID/1 -> Data Type Conversion7/1
  Data1/1 -> Data Type Conversion1/1
  Data2/1 -> Data Type Conversion2/1
  Data3/1 -> Data Type Conversion3/1
  Data4/1 -> Data Type Conversion4/1
  Data5/1 -> Data Type Conversion5/1
  Data6/1 -> Data Type Conversion6/1
  RollingCounter/1 -> Mux/8

== system Control_Test/Config/EmptySet1/Empty7 ==
  RollingCounter : Inport
  Data Type Conversion{1..7} (7 alike) : DataTypeConversion
  Data{1..6} (6 alike) : Constant  Value=0
  ID : Constant  Value=0
  Mux : Mux  Inputs=8
  PacketOut : Outport
  wires:
  Data Type Conversion7/1 -> Mux/1
  Data Type Conversion5/1 -> Mux/6
  Data Type Conversion3/1 -> Mux/4
  Data Type Conversion1/1 -> Mux/2
  Data Type Conversion2/1 -> Mux/3
  Data Type Conversion6/1 -> Mux/7
  Data Type Conversion4/1 -> Mux/5
  Mux/1 -> PacketOut/1
  ID/1 -> Data Type Conversion7/1
  Data1/1 -> Data Type Conversion1/1
  Data2/1 -> Data Type Conversion2/1
  Data3/1 -> Data Type Conversion3/1
  Data4/1 -> Data Type Conversion4/1
  Data5/1 -> Data Type Conversion5/1
  Data6/1 -> Data Type Conversion6/1
  RollingCounter/1 -> Mux/8

== system Control_Test/Config/EmptySet1/Empty8 ==
  RollingCounter : Inport
  Data Type Conversion{1..7} (7 alike) : DataTypeConversion
  Data{1..6} (6 alike) : Constant  Value=0
  ID : Constant  Value=0
  Mux : Mux  Inputs=8
  PacketOut : Outport
  wires:
  RollingCounter/1 -> Mux/8
  Data6/1 -> Data Type Conversion6/1
  Data5/1 -> Data Type Conversion5/1
  Data4/1 -> Data Type Conversion4/1
  Data3/1 -> Data Type Conversion3/1
  Data2/1 -> Data Type Conversion2/1
  Data1/1 -> Data Type Conversion1/1
  ID/1 -> Data Type Conversion7/1
  Mux/1 -> PacketOut/1
  Data Type Conversion4/1 -> Mux/5
  Data Type Conversion6/1 -> Mux/7
  Data Type Conversion2/1 -> Mux/3
  Data Type Conversion1/1 -> Mux/2
  Data Type Conversion3/1 -> Mux/4
  Data Type Conversion5/1 -> Mux/6
  Data Type Conversion7/1 -> Mux/1

== system Control_Test/Config/EmptySet2/Empty1 ==
  RollingCounter : Inport
  Data Type Conversion{1..7} (7 alike) : DataTypeConversion
  Data{1..6} (6 alike) : Constant  Value=0
  ID : Constant  Value=0
  Mux : Mux  Inputs=8
  PacketOut : Outport
  wires:
  Data Type Conversion7/1 -> Mux/1
  Data Type Conversion5/1 -> Mux/6
  Data Type Conversion3/1 -> Mux/4
  Data Type Conversion1/1 -> Mux/2
  Data Type Conversion2/1 -> Mux/3
  Data Type Conversion6/1 -> Mux/7
  Data Type Conversion4/1 -> Mux/5
  Mux/1 -> PacketOut/1
  ID/1 -> Data Type Conversion7/1
  Data1/1 -> Data Type Conversion1/1
  Data2/1 -> Data Type Conversion2/1
  Data3/1 -> Data Type Conversion3/1
  Data4/1 -> Data Type Conversion4/1
  Data5/1 -> Data Type Conversion5/1
  Data6/1 -> Data Type Conversion6/1
  RollingCounter/1 -> Mux/8

== system Control_Test/Config/EmptySet2/Empty2 ==
  RollingCounter : Inport
  Data Type Conversion{1..7} (7 alike) : DataTypeConversion
  Data{1..6} (6 alike) : Constant  Value=0
  ID : Constant  Value=0
  Mux : Mux  Inputs=8
  PacketOut : Outport
  wires:
  RollingCounter/1 -> Mux/8
  Data6/1 -> Data Type Conversion6/1
  Data5/1 -> Data Type Conversion5/1
  Data4/1 -> Data Type Conversion4/1
  Data3/1 -> Data Type Conversion3/1
  Data2/1 -> Data Type Conversion2/1
  Data1/1 -> Data Type Conversion1/1
  ID/1 -> Data Type Conversion7/1
  Mux/1 -> PacketOut/1
  Data Type Conversion4/1 -> Mux/5
  Data Type Conversion6/1 -> Mux/7
  Data Type Conversion2/1 -> Mux/3
  Data Type Conversion1/1 -> Mux/2
  Data Type Conversion3/1 -> Mux/4
  Data Type Conversion5/1 -> Mux/6
  Data Type Conversion7/1 -> Mux/1

== system Control_Test/Config/EmptySet2/Empty3 ==
  RollingCounter : Inport
  Data Type Conversion{1..7} (7 alike) : DataTypeConversion
  Data{1..6} (6 alike) : Constant  Value=0
  ID : Constant  Value=0
  Mux : Mux  Inputs=8
  PacketOut : Outport
  wires:
  RollingCounter/1 -> Mux/8
  Data6/1 -> Data Type Conversion6/1
  Data5/1 -> Data Type Conversion5/1
  Data4/1 -> Data Type Conversion4/1
  Data3/1 -> Data Type Conversion3/1
  Data2/1 -> Data Type Conversion2/1
  Data1/1 -> Data Type Conversion1/1
  ID/1 -> Data Type Conversion7/1
  Mux/1 -> PacketOut/1
  Data Type Conversion4/1 -> Mux/5
  Data Type Conversion6/1 -> Mux/7
  Data Type Conversion2/1 -> Mux/3
  Data Type Conversion1/1 -> Mux/2
  Data Type Conversion3/1 -> Mux/4
  Data Type Conversion5/1 -> Mux/6
  Data Type Conversion7/1 -> Mux/1

== system Control_Test/Config/EmptySet2/Empty4 ==
  RollingCounter : Inport
  Data Type Conversion{1..7} (7 alike) : DataTypeConversion
  Data{1..6} (6 alike) : Constant  Value=0
  ID : Constant  Value=0
  Mux : Mux  Inputs=8
  PacketOut : Outport
  wires:
  Data Type Conversion7/1 -> Mux/1
  Data Type Conversion5/1 -> Mux/6
  Data Type Conversion3/1 -> Mux/4
  Data Type Conversion1/1 -> Mux/2
  Data Type Conversion2/1 -> Mux/3
  Data Type Conversion6/1 -> Mux/7
  Data Type Conversion4/1 -> Mux/5
  Mux/1 -> PacketOut/1
  ID/1 -> Data Type Conversion7/1
  Data1/1 -> Data Type Conversion1/1
  Data2/1 -> Data Type Conversion2/1
  Data3/1 -> Data Type Conversion3/1
  Data4/1 -> Data Type Conversion4/1
  Data5/1 -> Data Type Conversion5/1
  Data6/1 -> Data Type Conversion6/1
  RollingCounter/1 -> Mux/8

== system Control_Test/Config/EmptySet2/Empty5 ==
  RollingCounter : Inport
  Data Type Conversion{1..7} (7 alike) : DataTypeConversion
  Data{1..6} (6 alike) : Constant  Value=0
  ID : Constant  Value=0
  Mux : Mux  Inputs=8
  PacketOut : Outport
  wires:
  RollingCounter/1 -> Mux/8
  Data6/1 -> Data Type Conversion6/1
  Data5/1 -> Data Type Conversion5/1
  Data4/1 -> Data Type Conversion4/1
  Data3/1 -> Data Type Conversion3/1
  Data2/1 -> Data Type Conversion2/1
  Data1/1 -> Data Type Conversion1/1
  ID/1 -> Data Type Conversion7/1
  Mux/1 -> PacketOut/1
  Data Type Conversion4/1 -> Mux/5
  Data Type Conversion6/1 -> Mux/7
  Data Type Conversion2/1 -> Mux/3
  Data Type Conversion1/1 -> Mux/2
  Data Type Conversion3/1 -> Mux/4
  Data Type Conversion5/1 -> Mux/6
  Data Type Conversion7/1 -> Mux/1

== system Control_Test/Config/EmptySet2/Empty6 ==
  RollingCounter : Inport
  Data Type Conversion{1..7} (7 alike) : DataTypeConversion
  Data{1..6} (6 alike) : Constant  Value=0
  ID : Constant  Value=0
  Mux : Mux  Inputs=8
  PacketOut : Outport
  wires:
  Data Type Conversion7/1 -> Mux/1
  Data Type Conversion5/1 -> Mux/6
  Data Type Conversion3/1 -> Mux/4
  Data Type Conversion1/1 -> Mux/2
  Data Type Conversion2/1 -> Mux/3
  Data Type Conversion6/1 -> Mux/7
  Data Type Conversion4/1 -> Mux/5
  Mux/1 -> PacketOut/1
  ID/1 -> Data Type Conversion7/1
  Data1/1 -> Data Type Conversion1/1
  Data2/1 -> Data Type Conversion2/1
  Data3/1 -> Data Type Conversion3/1
  Data4/1 -> Data Type Conversion4/1
  Data5/1 -> Data Type Conversion5/1
  Data6/1 -> Data Type Conversion6/1
  RollingCounter/1 -> Mux/8

== system Control_Test/Config/EmptySet2/Empty7 ==
  RollingCounter : Inport
  Data Type Conversion{1..7} (7 alike) : DataTypeConversion
  Data{1..6} (6 alike) : Constant  Value=0
  ID : Constant  Value=0
  Mux : Mux  Inputs=8
  PacketOut : Outport
  wires:
  Data Type Conversion7/1 -> Mux/1
  Data Type Conversion5/1 -> Mux/6
  Data Type Conversion3/1 -> Mux/4
  Data Type Conversion1/1 -> Mux/2
  Data Type Conversion2/1 -> Mux/3
  Data Type Conversion6/1 -> Mux/7
  Data Type Conversion4/1 -> Mux/5
  Mux/1 -> PacketOut/1
  ID/1 -> Data Type Conversion7/1
  Data1/1 -> Data Type Conversion1/1
  Data2/1 -> Data Type Conversion2/1
  Data3/1 -> Data Type Conversion3/1
  Data4/1 -> Data Type Conversion4/1
  Data5/1 -> Data Type Conversion5/1
  Data6/1 -> Data Type Conversion6/1
  RollingCounter/1 -> Mux/8

== system Control_Test/Config/EmptySet2/Empty8 ==
  RollingCounter : Inport
  Data Type Conversion{1..7} (7 alike) : DataTypeConversion
  Data{1..6} (6 alike) : Constant  Value=0
  ID : Constant  Value=0
  Mux : Mux  Inputs=8
  PacketOut : Outport
  wires:
  RollingCounter/1 -> Mux/8
  Data6/1 -> Data Type Conversion6/1
  Data5/1 -> Data Type Conversion5/1
  Data4/1 -> Data Type Conversion4/1
  Data3/1 -> Data Type Conversion3/1
  Data2/1 -> Data Type Conversion2/1
  Data1/1 -> Data Type Conversion1/1
  ID/1 -> Data Type Conversion7/1
  Mux/1 -> PacketOut/1
  Data Type Conversion4/1 -> Mux/5
  Data Type Conversion6/1 -> Mux/7
  Data Type Conversion2/1 -> Mux/3
  Data Type Conversion1/1 -> Mux/2
  Data Type Conversion3/1 -> Mux/4
  Data Type Conversion5/1 -> Mux/6
  Data Type Conversion7/1 -> Mux/1

== system Control_Test/Config/Set1/0x1011 ==
  note: 1.Data: number of config messages sent from the computer (minus this one)
      | 2.Data: number of continuous messages sent from the computer
  RollingCounter : Inport
  Data Type Conversion{,1..6} (7 alike) : DataTypeConversion
  Data1 : Constant  Value=39
  Data2 : Constant  Value=5
  Data3 : Constant  Value=8
  Data4 : Constant  Value=0
  Data5 : Constant  Value=0
  Data6 : Constant  Value=0
  ID : Constant  Value=0x1011
  Mux : Mux  Inputs=8
  PacketOut : Outport
  wires:
  Mux/1 -> PacketOut/1
  ID/1 -> Data Type Conversion6/1
  Data1/1 -> Data Type Conversion/1
  Data2/1 -> Data Type Conversion1/1
  Data3/1 -> Data Type Conversion2/1
  Data4/1 -> Data Type Conversion3/1
  Data5/1 -> Data Type Conversion4/1
  Data6/1 -> Data Type Conversion5/1
  RollingCounter/1 -> Mux/8
  Data Type Conversion1/1 -> Mux/3
  Data Type Conversion3/1 -> Mux/5
  Data Type Conversion5/1 -> Mux/7
  Data Type Conversion/1 -> Mux/2
  Data Type Conversion2/1 -> Mux/4
  Data Type Conversion4/1 -> Mux/6
  Data Type Conversion6/1 -> Mux/1

== system Control_Test/Config/Set1/Empty1 ==
  RollingCounter : Inport
  Data Type Conversion{1..7} (7 alike) : DataTypeConversion
  Data{1..6} (6 alike) : Constant  Value=0
  ID : Constant  Value=0
  Mux : Mux  Inputs=8
  PacketOut : Outport
  wires:
  RollingCounter/1 -> Mux/8
  Data6/1 -> Data Type Conversion6/1
  Data5/1 -> Data Type Conversion5/1
  Data4/1 -> Data Type Conversion4/1
  Data3/1 -> Data Type Conversion3/1
  Data2/1 -> Data Type Conversion2/1
  Data1/1 -> Data Type Conversion1/1
  ID/1 -> Data Type Conversion7/1
  Mux/1 -> PacketOut/1
  Data Type Conversion4/1 -> Mux/5
  Data Type Conversion6/1 -> Mux/7
  Data Type Conversion2/1 -> Mux/3
  Data Type Conversion1/1 -> Mux/2
  Data Type Conversion3/1 -> Mux/4
  Data Type Conversion5/1 -> Mux/6
  Data Type Conversion7/1 -> Mux/1

== system Control_Test/Config/Set1/Empty2 ==
  RollingCounter : Inport
  Data Type Conversion{1..7} (7 alike) : DataTypeConversion
  Data{1..6} (6 alike) : Constant  Value=0
  ID : Constant  Value=0
  Mux : Mux  Inputs=8
  PacketOut : Outport
  wires:
  Data Type Conversion7/1 -> Mux/1
  Data Type Conversion5/1 -> Mux/6
  Data Type Conversion3/1 -> Mux/4
  Data Type Conversion1/1 -> Mux/2
  Data Type Conversion2/1 -> Mux/3
  Data Type Conversion6/1 -> Mux/7
  Data Type Conversion4/1 -> Mux/5
  Mux/1 -> PacketOut/1
  ID/1 -> Data Type Conversion7/1
  Data1/1 -> Data Type Conversion1/1
  Data2/1 -> Data Type Conversion2/1
  Data3/1 -> Data Type Conversion3/1
  Data4/1 -> Data Type Conversion4/1
  Data5/1 -> Data Type Conversion5/1
  Data6/1 -> Data Type Conversion6/1
  RollingCounter/1 -> Mux/8

== system Control_Test/Config/Set1/Empty3 ==
  RollingCounter : Inport
  Data Type Conversion{1..7} (7 alike) : DataTypeConversion
  Data{1..6} (6 alike) : Constant  Value=0
  ID : Constant  Value=0
  Mux : Mux  Inputs=8
  PacketOut : Outport
  wires:
  RollingCounter/1 -> Mux/8
  Data6/1 -> Data Type Conversion6/1
  Data5/1 -> Data Type Conversion5/1
  Data4/1 -> Data Type Conversion4/1
  Data3/1 -> Data Type Conversion3/1
  Data2/1 -> Data Type Conversion2/1
  Data1/1 -> Data Type Conversion1/1
  ID/1 -> Data Type Conversion7/1
  Mux/1 -> PacketOut/1
  Data Type Conversion4/1 -> Mux/5
  Data Type Conversion6/1 -> Mux/7
  Data Type Conversion2/1 -> Mux/3
  Data Type Conversion1/1 -> Mux/2
  Data Type Conversion3/1 -> Mux/4
  Data Type Conversion5/1 -> Mux/6
  Data Type Conversion7/1 -> Mux/1

== system Control_Test/Config/Set1/Empty4 ==
  RollingCounter : Inport
  Data Type Conversion{1..7} (7 alike) : DataTypeConversion
  Data{1..6} (6 alike) : Constant  Value=0
  ID : Constant  Value=0
  Mux : Mux  Inputs=8
  PacketOut : Outport
  wires:
  Data Type Conversion7/1 -> Mux/1
  Data Type Conversion5/1 -> Mux/6
  Data Type Conversion3/1 -> Mux/4
  Data Type Conversion1/1 -> Mux/2
  Data Type Conversion2/1 -> Mux/3
  Data Type Conversion6/1 -> Mux/7
  Data Type Conversion4/1 -> Mux/5
  Mux/1 -> PacketOut/1
  ID/1 -> Data Type Conversion7/1
  Data1/1 -> Data Type Conversion1/1
  Data2/1 -> Data Type Conversion2/1
  Data3/1 -> Data Type Conversion3/1
  Data4/1 -> Data Type Conversion4/1
  Data5/1 -> Data Type Conversion5/1
  Data6/1 -> Data Type Conversion6/1
  RollingCounter/1 -> Mux/8

== system Control_Test/Config/Set1/Empty5 ==
  RollingCounter : Inport
  Data Type Conversion{1..7} (7 alike) : DataTypeConversion
  Data{1..6} (6 alike) : Constant  Value=0
  ID : Constant  Value=0
  Mux : Mux  Inputs=8
  PacketOut : Outport
  wires:
  RollingCounter/1 -> Mux/8
  Data6/1 -> Data Type Conversion6/1
  Data5/1 -> Data Type Conversion5/1
  Data4/1 -> Data Type Conversion4/1
  Data3/1 -> Data Type Conversion3/1
  Data2/1 -> Data Type Conversion2/1
  Data1/1 -> Data Type Conversion1/1
  ID/1 -> Data Type Conversion7/1
  Mux/1 -> PacketOut/1
  Data Type Conversion4/1 -> Mux/5
  Data Type Conversion6/1 -> Mux/7
  Data Type Conversion2/1 -> Mux/3
  Data Type Conversion1/1 -> Mux/2
  Data Type Conversion3/1 -> Mux/4
  Data Type Conversion5/1 -> Mux/6
  Data Type Conversion7/1 -> Mux/1

== system Control_Test/Config/Set1/Empty6 ==
  RollingCounter : Inport
  Data Type Conversion{1..7} (7 alike) : DataTypeConversion
  Data{1..6} (6 alike) : Constant  Value=0
  ID : Constant  Value=0
  Mux : Mux  Inputs=8
  PacketOut : Outport
  wires:
  Data Type Conversion7/1 -> Mux/1
  Data Type Conversion5/1 -> Mux/6
  Data Type Conversion3/1 -> Mux/4
  Data Type Conversion1/1 -> Mux/2
  Data Type Conversion2/1 -> Mux/3
  Data Type Conversion6/1 -> Mux/7
  Data Type Conversion4/1 -> Mux/5
  Mux/1 -> PacketOut/1
  ID/1 -> Data Type Conversion7/1
  Data1/1 -> Data Type Conversion1/1
  Data2/1 -> Data Type Conversion2/1
  Data3/1 -> Data Type Conversion3/1
  Data4/1 -> Data Type Conversion4/1
  Data5/1 -> Data Type Conversion5/1
  Data6/1 -> Data Type Conversion6/1
  RollingCounter/1 -> Mux/8

== system Control_Test/Config/Set1/Empty7 ==
  RollingCounter : Inport
  Data Type Conversion{1..7} (7 alike) : DataTypeConversion
  Data{1..6} (6 alike) : Constant  Value=0
  ID : Constant  Value=0
  Mux : Mux  Inputs=8
  PacketOut : Outport
  wires:
  RollingCounter/1 -> Mux/8
  Data6/1 -> Data Type Conversion6/1
  Data5/1 -> Data Type Conversion5/1
  Data4/1 -> Data Type Conversion4/1
  Data3/1 -> Data Type Conversion3/1
  Data2/1 -> Data Type Conversion2/1
  Data1/1 -> Data Type Conversion1/1
  ID/1 -> Data Type Conversion7/1
  Mux/1 -> PacketOut/1
  Data Type Conversion4/1 -> Mux/5
  Data Type Conversion6/1 -> Mux/7
  Data Type Conversion2/1 -> Mux/3
  Data Type Conversion1/1 -> Mux/2
  Data Type Conversion3/1 -> Mux/4
  Data Type Conversion5/1 -> Mux/6
  Data Type Conversion7/1 -> Mux/1
